simulink model "AC_base_1_VSM_2_22a"  (R2022a)
settings: Solver=ode3  StartTime=0.0  StopTime=8  FixedStep=HWSampleTime  RelTol=1e-3
undefined symbols (not defined in the file): ControlSampleTime, DiscIntNeverNeededParam, HWSampleTime, Ipwm_back, Ipwm_off, LCL, Manage, Oversample, Param, scaling_factor, SM, Ts, V_DC, VSMCTRL
libraries: fl_lib x100, nesl_utility x63, simulink x38, FriedrichLibrary x38, ee_lib x20, simulink_extras x14, TriphaseHardwaremodule x12, spsEdgeDetectorLib x2, StateMachines x2, slpidlib x2, spsPower3phInstantaneousLib x1
(part 5 of 7)

== system AC_base_1_VSM_2_22a/Variant Subsystem3/VSM/VSM1/VSM/CONTROL/VSMOC1 ==
  Manage : Inport
  Meas : Inport  Port=2
  u_inv_dq : Inport  Port=3
  Bus Selector1 : BusSelector  OutputSignals=enable_VSM.enable_ctrl,Param.VSM,enable_VSM.enable_inertia,sp_VSM
  Bus Selector11 : BusSelector  OutputSignals=phi
  Bus Selector2 : BusSelector  OutputSignals=PQ,PLL,u_cap.u_cap_dq0
  Selector : Selector  InputPortWidth=3  IndexOptions=Index vector (dialog)  Indices=[1 2]  OutputSizes=1
  Switch : Switch  Criteria=u2 ~= 0  SaturateOnIntegerOverflow=off  InputSameDT=off
  VSMOC : Subsystem
  phi_rad : Outport  VectorParamsAs1DForOutWhenUnconnected=off
  sp_u_inv_dq : Outport  Port=2  InitialOutput=[1 0]  VectorParamsAs1DForOutWhenUnconnected=off
  VSMdiag : Outport  Port=3  VectorParamsAs1DForOutWhenUnconnected=off
  wires:
  Bus Selector11/1 -> Switch/3  "<phi>"
  VSMOC/1(phi_rad) -> Switch/1
  VSMOC/3(VSMdiag) -> VSMdiag/1
  VSMOC/2(sp_u_inv_dq) -> sp_u_inv_dq/1
  Switch/1 -> phi_rad/1
  Manage/1 -> Bus Selector1/1
  Bus Selector1/1 -> VSMOC/Enable, Switch/2  "<enable_ctrl>"
  Meas/1 -> Bus Selector2/1
  Bus Selector2/2 -> VSMOC/5(PLL), Bus Selector11/1  "<PLL>"
  Bus Selector1/2 -> VSMOC/1(Param)  "<VSM>"
  Bus Selector1/3 -> VSMOC/2(enable_inertia)  "<enable_inertia>"
  Bus Selector1/4 -> VSMOC/3(sp_VSM)  "<sp_VSM>"
  u_inv_dq/1 -> VSMOC/6(u_inv_dq)
  Bus Selector2/3 -> Selector/1  "<u_cap_dq0>"
  Selector/1 -> VSMOC/7(u_cap_dq1)
  Bus Selector2/1 -> VSMOC/4(PQ_meas)  "<PQ>"

== system AC_base_1_VSM_2_22a/Variant Subsystem3/VSM/VSM1/VSM/CONTROL/Virtual Circuit mit R und L ==
  Param : Inport
  Reset : Inport  Port=2
  i_dq0 : Inport  Port=3
  Phi : Inport  Port=4
  Bus Selector : BusSelector  OutputSignals=R1,L1
  Bus Selector1 : BusSelector  OutputSignals=R1t,tauR,L1t,tauL
  Current Predictor : Subsystem  Commented=on
  L_Matrix : Gain  Gain=[0 -1 0;1 0 0; 0 0 0]
  L_Matrix1 : Gain  Gain=[0 -1 0;1 0 0; 0 0 0]
  PT1 : Subsystem  mask{K=1, Init=0, Ts=ControlSampleTime}
      mask prompts: K "Gain"; Init "Initial input"; Ts "Sample time"
      mask DialogControl DescGroupVar Prompt: PT1 discrete
      mask DialogControl DescTextVar Prompt: Simple discrete PT1
      mask Display:
      | text(0.5,0.5,get_param(gcb,'K'),'HorizontalAlignment','center','VerticalAlignment','Bottom')
      | text(0.5,0.5,'1 + s.tau','HorizontalAlignment','center','VerticalAlignment','Top')
      | plot([0.3 0.7],[0.5 0.5])
  PT2 : Subsystem  mask{K=1, Init=0, Ts=ControlSampleTime}
      mask prompts: K "Gain"; Init "Initial input"; Ts "Sample time"
      mask DialogControl DescGroupVar Prompt: PT1 discrete
      mask DialogControl DescTextVar Prompt: Simple discrete PT1
      mask Display:
      | text(0.5,0.5,get_param(gcb,'K'),'HorizontalAlignment','center','VerticalAlignment','Bottom')
      | text(0.5,0.5,'1 + s.tau','HorizontalAlignment','center','VerticalAlignment','Top')
      | plot([0.3 0.7],[0.5 0.5])
  "Param " : InportShadow
  Phi1 : InportShadow  Port=4
  Product : Product  Multiplication=Matrix(*)
  Product1 : Product  Multiplication=Matrix(*)
  Product2 : Product  Multiplication=Matrix(*)
  R_Matrix : Gain  Gain=[1 0 0;0 1 0; 0 0 0]
  R_Matrix1 : Gain  Gain=[1 0 0;0 1 0; 0 0 0]
  Reset1 : InportShadow  Port=2
  Sum : Sum  Inputs=++|
  Sum1 : Sum  Inputs=++|
  Sum2 : Sum  Inputs=|++
  " u_dq0" : Outport
  wires:
  Param/1 -> Bus Selector/1
  Bus Selector/1 -> R_Matrix/1  "<R1>"
  i_dq0/1 -> Product/2, PT2/1(U), PT1/1(U)
  Bus Selector/2 -> L_Matrix/1  "<L1>"
  L_Matrix/1 -> Sum/1
  R_Matrix/1 -> Sum/2
  Sum/1 -> Product/1
  "Param "/1 -> Bus Selector1/1
  R_Matrix1/1 -> Product1/1
  Product1/1 -> Sum1/1
  Bus Selector1/1 -> R_Matrix1/1  "<R1t>"
  Bus Selector1/4 -> PT2/2(tau)  "<tauL>"
  Bus Selector1/2 -> PT1/2(tau)  "<tauR>"
  Bus Selector1/3 -> L_Matrix1/1  "<L1t>"
  L_Matrix1/1 -> Product2/1
  Product2/1 -> Sum1/2
  Sum2/1 -> " u_dq0"/1
  PT1/1(Y) -> Product1/2
  Phi/1 -> PT1/4(Phi)
  Phi1/1 -> PT2/4(Phi)
  Reset/1 -> PT1/3(Reset)
  Reset1/1 -> PT2/3(Reset)
  PT2/1(Y) -> Product2/2
  Product/1 -> Sum2/1

== system AC_base_1_VSM_2_22a/Variant Subsystem3/VSM/VSM1/VSM/CONTROL/Virtual Circuit1 ==
  Param : Inport
  Reset : Inport  Port=2
  i_dq0 : Inport  Port=3
  Phi : Inport  Port=4
  Bus Selector : BusSelector  OutputSignals=R1,L1
  Bus Selector1 : BusSelector  OutputSignals=R1t,tauR,L1t,tauL
  Current Predictor : Subsystem  Commented=on
  L_Matrix : Gain  Gain=[0 -1 0;1 0 0; 0 0 0]
  L_Matrix1 : Gain  Gain=[0 -1 0;1 0 0; 0 0 0]
  PT1 : Subsystem  mask{K=1, Init=0, Ts=ControlSampleTime}
      mask prompts: K "Gain"; Init "Initial input"; Ts "Sample time"
      mask DialogControl DescGroupVar Prompt: PT1 discrete
      mask DialogControl DescTextVar Prompt: Simple discrete PT1
      mask Display:
      | text(0.5,0.5,get_param(gcb,'K'),'HorizontalAlignment','center','VerticalAlignment','Bottom')
      | text(0.5,0.5,'1 + s.tau','HorizontalAlignment','center','VerticalAlignment','Top')
      | plot([0.3 0.7],[0.5 0.5])
  PT2 : Subsystem  Commented=on  mask{K=1, Init=0, Ts=ControlSampleTime}
      mask prompts: K "Gain"; Init "Initial input"; Ts "Sample time"
      mask DialogControl DescGroupVar Prompt: PT1 discrete
      mask DialogControl DescTextVar Prompt: Simple discrete PT1
      mask Display:
      | text(0.5,0.5,get_param(gcb,'K'),'HorizontalAlignment','center','VerticalAlignment','Bottom')
      | text(0.5,0.5,'1 + s.tau','HorizontalAlignment','center','VerticalAlignment','Top')
      | plot([0.3 0.7],[0.5 0.5])
  "Param " : InportShadow
  Phi1 : InportShadow  Port=4
  Product : Product  Multiplication=Matrix(*)
  Product1 : Product  Multiplication=Matrix(*)
  Product2 : Product  Commented=on  Multiplication=Matrix(*)
  Product3 : Product  Multiplication=Matrix(*)
  R_Matrix : Gain  Gain=[1 0 0;0 1 0; 0 0 0]
  R_Matrix1 : Gain  Gain=[1 0 0;0 1 0; 0 0 0]
  Reset1 : InportShadow  Port=2
  Scope : Scope  NumInputPorts=2
  Scope1 : Scope
  Sum : Sum  Inputs=++|
  Sum1 : Sum  Inputs=++|
  Sum2 : Sum  Inputs=|++
  " u_dq0" : Outport
  wires:
  Param/1 -> Bus Selector/1
  Bus Selector/1 -> R_Matrix/1  "<R1>"
  i_dq0/1 -> PT2/1(U), PT1/1(U), Product3/2, Product/2
  Bus Selector/2 -> L_Matrix/1  "<L1>"
  L_Matrix/1 -> Sum/1
  R_Matrix/1 -> Product3/1, Sum/2
  Sum/1 -> Product/1
  "Param "/1 -> Bus Selector1/1
  Product/1 -> Sum2/1
  R_Matrix1/1 -> Product1/1
  Product1/1 -> Scope/2, Sum1/1
  Bus Selector1/1 -> R_Matrix1/1  "<R1t>"
  Bus Selector1/4 -> PT2/2(tau)  "<tauL>"
  Bus Selector1/2 -> PT1/2(tau)  "<tauR>"
  Bus Selector1/3 -> L_Matrix1/1  "<L1t>"
  L_Matrix1/1 -> Product2/1
  PT2/1(Y) -> Product2/2
  Product2/1 -> Scope1/1, Sum1/2
  Sum1/1 -> Sum2/2
  Sum2/1 -> " u_dq0"/1
  PT1/1(Y) -> Product1/2
  Phi1/1 -> PT2/4(Phi)
  Reset/1 -> PT1/3(Reset)
  Reset1/1 -> PT2/3(Reset)
  Product3/1 -> Scope/1

== system AC_base_1_VSM_2_22a/Variant Subsystem3/VSM/VSM1/VSM/CONTROL/active_damping ==
  enable_damp_dq : Inport
  Reset : Inport  Port=2
  u_dq0 : Inport  Port=3
  Phi : Inport  Port=4
  Bus Selector : BusSelector  OutputSignals=Damp_dq,Damp_dq,Damp_CM,OmLead,OmLag
  Integrator (inertia) : DiscreteIntegrator  gainval=1  ExternalReset=rising  InitialConditionSource=external  InitialCondition=1  SampleTime=ControlSampleTime  ICPrevOutput=DiscIntNeverNeededParam  ICPrevScaledInput=DiscIntNeverNeededParam
  Mux : Mux  Inputs=3
  Product{,1..3} (4 alike) : Product
  Sum : Sum  Inputs=|+-
  Sum2 : Sum  Inputs=++|
  Unit Delay2 : UnitDelay  InitialCondition=[0 0 0]  SampleTime=ControlSampleTime  HasFrameUpgradeWarning=on
  dq0->ab0 phi : FriedrichLibrary/Transformations/dq0->ab0 phi  SystemSampleTime=-1  VariantActivationTime=update diagram  Latency=0  AutoFrameSizeCalculation=off
  damp_dq0 : Outport  VectorParamsAs1DForOutWhenUnconnected=off
  wires:
  Product2/1 -> Sum/1
  Integrator (inertia)/1 -> Unit Delay2/1, Sum2/2
  Product3/1 -> Sum/2
  Sum2/1 -> Product3/1, Product1/2
  Sum/1 -> Integrator (inertia)/1
  enable_damp_dq/1 -> Bus Selector/1
  Bus Selector/1 -> Mux/1  "<Damp_dq>"
  Bus Selector/2 -> Mux/2  "<Damp_dq>"
  Bus Selector/3 -> Mux/3  "<Damp_CM>"
  u_dq0/1 -> Product/2
  Product/1 -> Sum2/1, Product2/2
  Mux/1 -> Product1/1, Product/1  "enable"
  Product1/1 -> damp_dq0/1
  Phi/1 -> dq0->ab0 phi/2
  Reset/1 -> Integrator (inertia)/2
  Unit Delay2/1 -> dq0->ab0 phi/1
  dq0->ab0 phi/1 -> Integrator (inertia)/3
  Bus Selector/4 -> Product2/1  "<OmLead>"
  Bus Selector/5 -> Product3/2  "<OmLag>"

== system AC_base_1_VSM_2_22a/Variant Subsystem3/VSM/VSM1/VSM/CONTROL/dq0 to duty ==
  phi_rad : Inport
  u_dq0 : Inport  Port=2
  u_dc : Inport  Port=3
  Bias : Bias  Bias=Ctrl.PWM.tauT*Ctrl.PU.omegab  SaturateOnIntegerOverflow=off
  Bus Creator3 : BusCreator  Inputs=2
  Divide : Product  Inputs=*/
  Gain : Gain  Gain=eye(NrChannels,3)  Multiplication=Matrix(K*u)
  Modulation : FriedrichLibrary/Transformations/Modulation  Method=Sine Modulation  Ts=ControlSampleTime
  SMA : FriedrichLibrary/Discrete Stuff/SMA  n_samples=1/ControlSampleTime/100  init_out=0
  Saturation : Saturate  UpperLimit=inf  LowerLimit=1
  Signal Specification1 : SignalSpecification
  dq0->ab0 phi : FriedrichLibrary/Transformations/dq0->ab0 phi  SystemSampleTime=-1  VariantActivationTime=update diagram  Latency=0  AutoFrameSizeCalculation=off
  d : Outport  VectorParamsAs1DForOutWhenUnconnected=off
  pwmDiag : Outport  Port=2  VectorParamsAs1DForOutWhenUnconnected=off
  wires:
  phi_rad/1 -> Bus Creator3/2, Bias/1  "phi"
  u_dq0/1 -> dq0->ab0 phi/1
  Divide/1 -> Modulation/1  "ab0 norm"
  dq0->ab0 phi/1 -> Divide/1
  Modulation/1 -> Gain/1
  Bias/1 -> dq0->ab0 phi/2
  u_dc/1 -> Saturation/1
  Bus Creator3/1 -> pwmDiag/1  "pwmDiag"
  Gain/1 -> Bus Creator3/1, Signal Specification1/1  "pwm"
  Signal Specification1/1 -> d/1
  Saturation/1 -> SMA/1
  SMA/1 -> Divide/2

== system AC_base_1_VSM_2_22a/Variant Subsystem3/VSM/VSM1/VSM/CONTROL/i_dq_ctrl ==
  note: Inrouting
  note: Outrouting
  note: PI Control
  Param : Inport
  enable_cc : Inport  Port=2
  sp_cc : Inport  Port=3
  ms_i_inv_dq : Inport  Port=4
  u_ff_dq : Inport  Port=5
  u_inv_dq : Inport  Port=6
  Enable : EnablePort  StatesWhenEnabling=reset
  Bus Creator2 : BusCreator  Inputs=4
  Bus Selector13 : BusSelector  OutputSignals=init_u_inv
  Constant : Constant
  Demux : Demux  Outputs=2
  From1 : From  Commented=on  GotoTag=initU
  Gain1 : Gain  Commented=on  Gain=Kff
  Gain2 : Gain  Gain=L_inv
  Gain4 : Gain  Gain=[0 -1;1 0]  Multiplication=Matrix(K*u)
  Gain5 : Gain  Commented=on  Gain=1-Kff
  Mux : Mux  Inputs=2
  PI : Subsystem
  Product : Product
  Product1 : Product
  Product2 : Product
  Scope : Scope  NumInputPorts=3
  Step : Step  Time=8  Before=1  After=0  SampleTime=0
  Sum1 : Sum  Inputs=+++
  Sum2 : Sum  Commented=on  Inputs=|+-
  Sum3 : Sum  Inputs=|+-
  Switch1 : Switch  Commented=on  Criteria=u2 > Threshold  SaturateOnIntegerOverflow=off  InputSameDT=off
  sp_u_inv_dq : Outport  VectorParamsAs1DForOutWhenUnconnected=off
  CCdiag : Outport  Port=2  VectorParamsAs1DForOutWhenUnconnected=off
  wires:
  Switch1/1 -> Sum2/1
  Gain4/1 -> Gain2/1
  Gain2/1 -> Sum2/2  "dq decouple"
  From1/1 -> Switch1/2
  Sum1/1 -> Scope/1, Product/2
  u_inv_dq/1 -> Switch1/1
  [Enable] -> PI/Enable
  Sum3/1 -> Demux/1
  sp_cc/1 -> [sp_i_dq], Sum3/1
  Param/1 -> Bus Selector13/1
  Bus Selector13/1 -> [initU]  "<init_u_inv>"
  [Enable] -> Product/1
  [sp_u_dq] -> Bus Creator2/3  "sp_u_dq"
  enable_cc/1 -> [Enable]  "enable_cc"
  [Enable] -> Bus Creator2/4  "enable_cc"
  Bus Creator2/1 -> CCdiag/1
  [sp_i_dq] -> Bus Creator2/1  "sp_i_dq"
  [i_dq] -> Bus Creator2/2  "i_dq"
  u_ff_dq/1 -> Scope/2, PI/2(u0), Gain1/1, Gain5/1
  Gain5/1 -> Switch1/3
  Product/1 -> sp_u_inv_dq/1, [sp_u_dq]
  ms_i_inv_dq/1 -> [i_dq], Sum3/2, Gain4/1
  Mux/1 -> PI/1(di)
  Demux/2 -> Product1/1
  Product1/1 -> Mux/2
  Product2/1 -> Mux/1
  Demux/1 -> Product2/1
  Constant/1 -> Product2/2, Product1/2
  PI/1(u) -> Sum1/1  "pi"

== system AC_base_1_VSM_2_22a/Variant Subsystem3/VSM/VSM1/VSM/MANAGEMENT/Subsystem1 ==
  i_inv_ab : Inport
  <i_inv_dq0> : Inport  Port=2
  <u_cap_ab0> : Inport  Port=3
  <PQ_out> : Inport  Port=4
  enable : Inport  Port=5
  i_out_ab : Inport  Port=6
  "AL brechen AL nicht mit FCN lösbar " : Memory
  Compare To Constant : simulink/Logic and Bit Operations/Compare To Constant  relop===  const=0  OutDataTypeStr=boolean
  Complex to Magnitude-Angle : ComplexToMagnitudeAngle
  Demux : Demux  Outputs=2
  Divide : Product  Inputs=*/
  Enabled Subsystem : Subsystem  TreatAsAtomicUnit=on
  Math Function1 : Math  Operator=square  SignedPower=on
  Math Function2 : Math  Operator=square  SignedPower=on
  Math Function3 : Math  Operator=square  SignedPower=on
  Max : MinMax  Function=max  Inputs=2
  Real-Imag to Complex : RealImagToComplex
  Scope : Scope  NumInputPorts=2
  Selector2 : Selector  InputPortWidth=3  IndexOptions=Index vector (dialog)  Indices=[1 2]  OutputSizes=1
  Sqrt1 : Sqrt
  Sqrt2 : Sqrt
  Sqrt3 : Sqrt
  Subsystem : Subsystem
  Sum of Elements1 : Sum  Inputs=+
  Sum of Elements2 : Sum  Inputs=+
  Sum of Elements3 : Sum  Inputs=+
  Transport Delay : TransportDelay  DelayTime=0.1
  Transport Delay1 : TransportDelay  DelayTime=0.1
  Unit Delay : UnitDelay  SampleTime=ControlSampleTime  HasFrameUpgradeWarning=on
  Unit Delay1 : UnitDelay  SampleTime=ControlSampleTime  HasFrameUpgradeWarning=on
  CC : Outport
  sp_CC : Outport  Port=2
  wires:
  Sum of Elements1/1 -> Sqrt2/1
  Selector2/1 -> Math Function2/1
  Math Function1/1 -> Sum of Elements1/1
  Sum of Elements2/1 -> Sqrt1/1
  "AL brechen AL nicht mit FCN lösbar "/1 -> Subsystem/1(i_inv)
  Sqrt1/1 -> Subsystem/4(U_cap), Divide/2
  Math Function2/1 -> Sum of Elements2/1
  <u_cap_ab0>/1 -> Selector2/1
  <i_inv_dq0>/1 -> "AL brechen AL nicht mit FCN lösbar "/1
  Subsystem/1(i_sp) -> sp_CC/1  "sp_CC"
  i_inv_ab/1 -> Math Function1/1
  Subsystem/2(CC) -> CC/1
  <PQ_out>/1 -> Divide/1, Subsystem/2(PQ_out)
  enable/1 -> Subsystem/Enable
  Compare To Constant/1 -> Enabled Subsystem/Enable
  Enabled Subsystem/1(i abs_pre) -> Scope/1, Unit Delay/1
  Subsystem/3(set) -> Compare To Constant/1
  Transport Delay/1 -> Enabled Subsystem/1(i_abs)
  Unit Delay/1 -> Subsystem/6(i abs_pre)
  Enabled Subsystem/2(i_pq_pre) -> Unit Delay1/1, Scope/2
  Unit Delay1/1 -> Subsystem/5(PQ_pre)
  Transport Delay1/1 -> Enabled Subsystem/2(i_pq)
  Math Function3/1 -> Sum of Elements3/1
  Sum of Elements3/1 -> Sqrt3/1
  i_out_ab/1 -> Math Function3/1
  Sqrt3/1 -> Max/1
  Sqrt2/1 -> Max/2, Transport Delay/1
  Max/1 -> Subsystem/3(iabs)
  Demux/1 -> Real-Imag to Complex/1
  Demux/2 -> Real-Imag to Complex/2
  Divide/1 -> Demux/1, Transport Delay1/1
  Real-Imag to Complex/1 -> Complex to Magnitude-Angle/1
  Complex to Magnitude-Angle/2 -> Subsystem/7(angle_i)

== system AC_base_1_VSM_2_22a/Variant Subsystem3/VSM/VSM1/VSM/MANAGEMENT/current_watchdog ==
  |i| set : Inport
  |i| reset : Inport  Port=2
  i_ab : Inport  Port=3
  sp_gain : Inport  Port=4
  PQ : Inport  Port=5
  i_inv : Inport  Port=6
  active_current_watchdog : EnablePort  StatesWhenEnabling=reset
  Divide : Product  Inputs=/**
  MATLAB Function : MATLAB Function  Commented=on  TreatAsAtomicUnit=on
  Math Function1 : Math  Operator=square  SignedPower=on
  Math Function2 : Math  Operator=square  SignedPower=on
  Math Function3 : Math  Operator=square  SignedPower=on
  Relational Operator : RelationalOperator  Operator=<=  OutDataTypeStr=boolean  InputSameDT=off
  Relational Operator1 : RelationalOperator  Operator=<=  OutDataTypeStr=boolean  InputSameDT=off
  S-R Flip-Flop1 : simulink_extras/Flip Flops/S-R Flip-Flop  initial_condition=0
  Scope : Scope  NumInputPorts=3
  Scope1 : Scope
  Sum of Elements1 : Sum  Inputs=+
  Terminator1 : Terminator
  enable_cc : Outport  VectorParamsAs1DForOutWhenUnconnected=off
  sp_gain_wd : Outport  Port=2  VectorParamsAs1DForOutWhenUnconnected=off
  wires:
  Math Function2/1 -> Relational Operator/1, MATLAB Function/2(set)
  i_ab/1 -> Math Function1/1
  Sum of Elements1/1 -> Relational Operator1/1, MATLAB Function/1(abs), Relational Operator/2
  Math Function1/1 -> Sum of Elements1/1
  Relational Operator1/1 -> S-R Flip-Flop1/2
  S-R Flip-Flop1/2 -> Terminator1/1
  Math Function3/1 -> Relational Operator1/2
  |i| reset/1 -> Divide/2, Math Function3/1
  |i| set/1 -> Divide/1, Math Function2/1
  sp_gain/1 -> Divide/3
  MATLAB Function/1(CC) -> enable_cc/1, Scope/1
  MATLAB Function/2(i) -> sp_gain_wd/1
  PQ/1 -> Scope1/1, MATLAB Function/3(p)
  i_inv/1 -> MATLAB Function/4(i_inv)

== system AC_base_1_VSM_2_22a/Variant Subsystem3/VSM/VSM1/VSM/MANAGEMENT/sp_VSM ==
  EnableRateLimit : Inport
  CMD : Inport  Port=2
  MEAS : Inport  Port=3
  Bus Creator : BusCreator  Inputs=3
  Bus Selector1 : BusSelector  OutputSignals=u_out.u_out_ab0
  Bus Selector6 : BusSelector  OutputSignals=Param.VSM.sp_f,Param.VSM.sp_E,Param.VSM.sp_PQ,Param.VSM.sp_PQ_limit
  "CMD " : InportShadow  Port=2
  E(PQ) : Subsystem
  PQ(U) Limit : Subsystem
  RateLimit : Subsystem
  Saturation : Saturate  UpperLimit=1  LowerLimit=-1
  sp_VSM : Outport  VectorParamsAs1DForOutWhenUnconnected=off
  wires:
  E(PQ)/1(sp_E) -> Bus Creator/2  "sp_E"
  Bus Selector6/2 -> E(PQ)/1(E)  "<sp_E>"
  Bus Selector6/3 -> Saturation/1  "<sp_PQ>"
  EnableRateLimit/1 -> RateLimit/Enable  "ENABLED"
  RateLimit/1(PQslow) -> E(PQ)/3(sp_PQ), PQ(U) Limit/1(sp_PQ)
  Bus Selector1/1 -> PQ(U) Limit/3(u_out)  "<u_out_ab0>"
  Bus Selector6/4 -> PQ(U) Limit/2(enable)  "<sp_PQ_limit>"
  PQ(U) Limit/1(sp_PQ_limit) -> Bus Creator/3  "sp_PQ"
  CMD/1 -> Bus Selector6/1
  MEAS/1 -> Bus Selector1/1
  Bus Selector6/1 -> Bus Creator/1  "<sp_f>"
  Bus Creator/1 -> sp_VSM/1
  "CMD "/1 -> E(PQ)/2(cmd)
  Saturation/1 -> RateLimit/1(PQ)

== system AC_base_1_VSM_2_22a/Variant Subsystem3/VSM/VSM1/VSM/Meas/SI -> pu ==
  MeasIn : Inport
  Bus Creator1 : BusCreator  Inputs=5
  Bus Selector : BusSelector  OutputSignals=meas_u_out,meas_i_out,meas_i_inverter,meas_u_dc,meas_u_cap
  Normalize : Gain  Gain=1/PU.Ub  OutDataTypeStr=double  RndMeth=Round
  Normalize1 : Gain  Gain=1/PU.Ib  OutDataTypeStr=double  RndMeth=Round
  Normalize2 : Gain  Gain=1/PU.Ib  OutDataTypeStr=double  RndMeth=Round
  Normalize3 : Gain  Gain=1/PU.Ub  OutDataTypeStr=double  RndMeth=Round
  Normalize4 : Gain  Gain=1/PU.Ub/2  OutDataTypeStr=double  RndMeth=Round
  MeasOut : Outport  VectorParamsAs1DForOutWhenUnconnected=off
  wires:
  Normalize3/1 -> Bus Creator1/5  "meas_u_cap"
  Bus Selector/5 -> Normalize3/1  "<meas_u_cap>"
  Bus Selector/4 -> Normalize4/1  "<meas_u_dc>"
  Bus Selector/3 -> Normalize1/1  "<meas_i_inverter>"
  Bus Selector/2 -> Normalize2/1  "<meas_i_out>"
  Bus Selector/1 -> Normalize/1  "<meas_u_out>"
  Bus Creator1/1 -> MeasOut/1
  Normalize4/1 -> Bus Creator1/4  "meas_vol_dc"
  Normalize2/1 -> Bus Creator1/2  "meas_i_out"
  Normalize1/1 -> Bus Creator1/3  "meas_i_inverter"
  Normalize/1 -> Bus Creator1/1  "meas_u_out"
  MeasIn/1 -> Bus Selector/1

== system AC_base_1_VSM_2_22a/Variant Subsystem3/VSM/VSM1/VSM/Meas/meas_i_inv ==
  abc : Inport
  phi : Inport  Port=2
  Bus Creator1 : BusCreator  Inputs=3
  PhN->ab2 : FriedrichLibrary/Transformations/PhN->ab0  SystemSampleTime=-1  VariantActivationTime=update diagram  Latency=0  AutoFrameSizeCalculation=off
  ab0->dq0-faster : FriedrichLibrary/Transformations/ab0->dq0-faster  SystemSampleTime=-1  VariantActivationTime=update diagram  Latency=0  AutoFrameSizeCalculation=off
  i_inv_x : Outport  VectorParamsAs1DForOutWhenUnconnected=off
  wires:
  ab0->dq0-faster/1 -> Bus Creator1/3  "i_inv_dq0"
  PhN->ab2/1 -> Bus Creator1/2, ab0->dq0-faster/1  "i_inv_ab0"
  abc/1 -> Bus Creator1/1, PhN->ab2/1  "i_inv_abc"
  phi/1 -> ab0->dq0-faster/2
  Bus Creator1/1 -> i_inv_x/1

== system AC_base_1_VSM_2_22a/Variant Subsystem3/VSM/VSM1/VSM/Meas/meas_i_out ==
  abc : Inport
  phi : Inport  Port=2
  Bus Creator1 : BusCreator  Inputs=3
  PhN->ab2 : FriedrichLibrary/Transformations/PhN->ab0  SystemSampleTime=-1  VariantActivationTime=update diagram  Latency=0  AutoFrameSizeCalculation=off
  ab0->dq0-faster : FriedrichLibrary/Transformations/ab0->dq0-faster  SystemSampleTime=-1  VariantActivationTime=update diagram  Latency=0  AutoFrameSizeCalculation=off
  i_out_x : Outport  VectorParamsAs1DForOutWhenUnconnected=off
  wires:
  ab0->dq0-faster/1 -> Bus Creator1/3  "i_out_dq0"
  PhN->ab2/1 -> Bus Creator1/2, ab0->dq0-faster/1  "i_out_ab0"
  abc/1 -> Bus Creator1/1, PhN->ab2/1  "i_out_abc"
  phi/1 -> ab0->dq0-faster/2
  Bus Creator1/1 -> i_out_x/1

== system AC_base_1_VSM_2_22a/Variant Subsystem3/VSM/VSM1/VSM/Meas/meas_u_cap ==
  abc : Inport
  phi : Inport  Port=2
  Bus Creator1 : BusCreator  Inputs=3
  PhN->ab2 : FriedrichLibrary/Transformations/PhN->ab0  SystemSampleTime=-1  VariantActivationTime=update diagram  Latency=0  AutoFrameSizeCalculation=off
  ab0->dq0-faster : FriedrichLibrary/Transformations/ab0->dq0-faster  SystemSampleTime=-1  VariantActivationTime=update diagram  Latency=0  AutoFrameSizeCalculation=off
  u_cap_x : Outport  VectorParamsAs1DForOutWhenUnconnected=off
  wires:
  Bus Creator1/1 -> u_cap_x/1
  phi/1 -> ab0->dq0-faster/2
  abc/1 -> PhN->ab2/1, Bus Creator1/1  "u_cap_abc"
  PhN->ab2/1 -> ab0->dq0-faster/1, Bus Creator1/2  "u_cap_ab0"
  ab0->dq0-faster/1 -> Bus Creator1/3  "u_cap_dq0"

== system AC_base_1_VSM_2_22a/Variant Subsystem3/VSM/VSM1/VSM/Meas/meas_u_out ==
  abc : Inport
  phi : Inport  Port=2
  Bus Creator1 : BusCreator  Inputs=3
  PhN->ab2 : FriedrichLibrary/Transformations/PhN->ab0  SystemSampleTime=-1  VariantActivationTime=update diagram  Latency=0  AutoFrameSizeCalculation=off
  ab0->dq0-faster : FriedrichLibrary/Transformations/ab0->dq0-faster  SystemSampleTime=-1  VariantActivationTime=update diagram  Latency=0  AutoFrameSizeCalculation=off
  u_out_x : Outport  VectorParamsAs1DForOutWhenUnconnected=off
  wires:
  Bus Creator1/1 -> u_out_x/1
  phi/1 -> ab0->dq0-faster/2
  abc/1 -> PhN->ab2/1, Bus Creator1/1  "u_out_abc"
  PhN->ab2/1 -> ab0->dq0-faster/1, Bus Creator1/2  "u_out_ab0"
  ab0->dq0-faster/1 -> Bus Creator1/3  "u_out_dq0"

== system AC_base_1_VSM_2_22a/Variant Subsystem3/VSM/VSM1/command_center/cmd_VSM/Current Control ==
  note: else: init with u cap
  Bus Creator6 : BusCreator  Inputs=5
  Bus Creator7 : BusCreator  Inputs=3
  Init with u_inv [0/1] : Constant  Value=VSMCTRL.CC.init_uinv
  activate : Constant  Value=VSMCTRL.CC.activate
  external_stop_cc1 : Constant  Value=0
  external_stop_cc4 : Constant  Value=0
  i_reset_abs : Constant  Value=VSMCTRL.CC.i_reset
  i_set_abs : Constant  Value=VSMCTRL.CC.i_set
  i_sp_gain : Constant  Value=VSMCTRL.CC.i_sp_gain
  Current Control : Outport  VectorParamsAs1DForOutWhenUnconnected=off
  wires:
  activate/1 -> Bus Creator7/1  "activate"
  i_reset_abs/1 -> Bus Creator7/3  "abs_i_reset"
  Bus Creator7/1 -> Bus Creator6/5  "watchdog"
  external_stop_cc4/1 -> Bus Creator6/2  "ex_start_cc"
  i_set_abs/1 -> Bus Creator7/2  "abs_i_set"
  i_sp_gain/1 -> Bus Creator6/4  "i_sp_gain"
  external_stop_cc1/1 -> Bus Creator6/3  "ex_stop_cc"
  Init with u_inv [0/1]/1 -> Bus Creator6/1  "init_u_inv"
  Bus Creator6/1 -> Current Control/1  "CC"

== system AC_base_1_VSM_2_22a/Variant Subsystem3/VSM/VSM1/command_center/cmd_VSM/Damping ==
  Bus Creator5 : BusCreator  Inputs=4
  EnableDamp_CM [0/1] : Constant  Value=VSMCTRL.VTFF.EnableCM
  EnableDamp_dq [0/1] : Constant  Value=VSMCTRL.VTFF.EnableDQ
  Omega Lag : Constant  Value=VSMCTRL.VTFF.OmLag
  Omega Lead : Constant  Value=VSMCTRL.VTFF.OmLead
  Damping : Outport  VectorParamsAs1DForOutWhenUnconnected=off
  wires:
  EnableDamp_CM [0/1]/1 -> Bus Creator5/2  "Damp_CM"
  EnableDamp_dq [0/1]/1 -> Bus Creator5/1  "Damp_dq"
  Bus Creator5/1 -> Damping/1
  Omega Lead/1 -> Bus Creator5/3  "OmLead"
  Omega Lag/1 -> Bus Creator5/4  "OmLag"

== system AC_base_1_VSM_2_22a/Variant Subsystem3/VSM/VSM1/command_center/cmd_VSM/Manage ==
  Bus Creator : BusCreator  Inputs=2
  connect : Constant
  enable : Constant
  Manage : Outport  VectorParamsAs1DForOutWhenUnconnected=off
  wires:
  Bus Creator/1 -> Manage/1
  connect/1 -> Bus Creator/1  "connect"
  enable/1 -> Bus Creator/2  "enable"

== system AC_base_1_VSM_2_22a/Variant Subsystem3/VSM/VSM1/command_center/cmd_VSM/Virtual Circuit ==
  Bus Creator9 : BusCreator  Inputs=7
  Virtual L1 : Constant  Value=VSMCTRL.VC.L1
  Virtual L1t : Constant  Value=VSMCTRL.VC.L1t
  Virtual R1 : Constant  Value=VSMCTRL.VC.R1
  Virtual R1t : Constant  Value=VSMCTRL.VC.R1t
  tau HP Slow : Constant  Value=VSMCTRL.VC.tauSlow
  tau Virtual L1 : Constant  Value=VSMCTRL.VC.tauL
  tau Virtual R1 : Constant  Value=VSMCTRL.VC.tauR
  Virtual Circuit : Outport  VectorParamsAs1DForOutWhenUnconnected=off
  wires:
  Virtual R1/1 -> Bus Creator9/1  "R1"
  Virtual R1t/1 -> Bus Creator9/2  "R1t"
  Virtual L1t/1 -> Bus Creator9/4  "L1t"
  Bus Creator9/1 -> Virtual Circuit/1
  Virtual L1/1 -> Bus Creator9/3  "L1"
  tau Virtual R1/1 -> Bus Creator9/5  "tauR"
  tau Virtual L1/1 -> Bus Creator9/6  "tauL"
  tau HP Slow/1 -> Bus Creator9/7  "tauS"

== system AC_base_1_VSM_2_22a/Variant Subsystem3/VSM/VSM1/command_center/cmd_VSM/Virtual Synchronous Machine ==
  note: 0 Dekaktiviert Init Tiefpass
  note: 0 Dekaktiviert Init Tiefpass
  Bus Creator3 : BusCreator  Inputs=12
  E(sp_PQ) : Constant  Value=VSMCTRL.SP.E_comp
  Ta : Constant  Value=VSMCTRL.VSM.Ta
  Ta1 : Constant  Value=VSMCTRL.VSM.kpf
  Ta2 : Constant  Value=VSMCTRL.VSM.kdf
  Ta3 : Constant  Value=VSMCTRL.VSM.ku
  Ta4 : Constant  Value=VSMCTRL.VSM.Tu
  Ta5 : Constant  Value=0
  Ta6 : Constant  Value=0
  sp_E [pu] : Constant  Value=VSMCTRL.SP.E
  sp_PQ [pu] : Constant  Value=VSMCTRL.SP.PQ
  sp_PQ(U) limit : Constant  Value=VSMCTRL.SP.PQU_lim
  sp_f [Hz] : Constant  Value=VSMCTRL.SP.f
  Virtual Synchronous Machine : Outport  VectorParamsAs1DForOutWhenUnconnected=off
  wires:
  sp_E [pu]/1 -> Bus Creator3/10  "sp_E"
  sp_PQ [pu]/1 -> Bus Creator3/9  "sp_PQ"
  sp_f [Hz]/1 -> Bus Creator3/8  "sp_f"
  sp_PQ(U) limit/1 -> Bus Creator3/11  "sp_PQ_limit"
  Ta/1 -> Bus Creator3/1  "Ta"
  Bus Creator3/1 -> Virtual Synchronous Machine/1
  Ta4/1 -> Bus Creator3/5  "Tu"
  Ta3/1 -> Bus Creator3/4  "ku"
  Ta2/1 -> Bus Creator3/3  "kdf"
  Ta1/1 -> Bus Creator3/2  "kpf"
  Ta6/1 -> Bus Creator3/7  "TPinit"
  Ta5/1 -> Bus Creator3/6  "Tuinit"
  E(sp_PQ)/1 -> Bus Creator3/12  "sp_E_comp"

== system AC_base_1_VSM_2_22a/Variant Subsystem1/VSM/Inverter AverageMdl LC SimScape2/Modul F30 fixed DC voltage Average SimScape/simscape_bridgefilter_aca/PWM Blocking1/Trigger Spike at new Control Sample ==
  Add : Sum  Inputs=+-
  Compare To Constant : simulink/Logic and Bit Operations/Compare To Constant  relop=~=  const=0  OutDataTypeStr=boolean
  Rate Transition : RateTransition  OutPortSampleTime=ControlSampleTime
  Rate Transition1 : RateTransition  OutPortSampleTime=ControlSampleTime
  Rate Transition2 : RateTransition  OutPortSampleTime=ControlSampleTime/Oversample
  S-R Flip-Flop1 : simulink_extras/Flip Flops/S-R Flip-Flop  initial_condition=1
  Unit Delay : UnitDelay  SampleTime=-1  HasFrameUpgradeWarning=on
  Unit Delay2 : UnitDelay  SampleTime=-1  HasFrameUpgradeWarning=on
  Unit Delay3 : UnitDelay  SampleTime=-1  HasFrameUpgradeWarning=on
  y : Outport
  wires:
  Rate Transition1/1 -> Unit Delay2/1
  Rate Transition/1 -> Unit Delay/1
  Unit Delay/1 -> S-R Flip-Flop1/2
  Add/1 -> Compare To Constant/1
  Compare To Constant/1 -> y/1
  Unit Delay3/1 -> Add/1
  Unit Delay2/1 -> S-R Flip-Flop1/1
  S-R Flip-Flop1/2 -> Rate Transition1/1
  Rate Transition2/1 -> Unit Delay3/1, Add/2
  S-R Flip-Flop1/1 -> Rate Transition/1, Rate Transition2/1

== system AC_base_1_VSM_2_22a/Variant Subsystem1/VSM/Inverter AverageMdl LC SimScape2/Modul F30 fixed DC voltage Average SimScape/simscape_bridgefilter_aca1/PWM Blocking1/Trigger Spike at new Control Sample ==
  Add : Sum  Inputs=+-
  Compare To Constant : simulink/Logic and Bit Operations/Compare To Constant  relop=~=  const=0  OutDataTypeStr=boolean
  Rate Transition : RateTransition  OutPortSampleTime=ControlSampleTime
  Rate Transition1 : RateTransition  OutPortSampleTime=ControlSampleTime
  Rate Transition2 : RateTransition  OutPortSampleTime=ControlSampleTime/Oversample
  S-R Flip-Flop1 : simulink_extras/Flip Flops/S-R Flip-Flop  initial_condition=1
  Unit Delay : UnitDelay  SampleTime=-1  HasFrameUpgradeWarning=on
  Unit Delay2 : UnitDelay  SampleTime=-1  HasFrameUpgradeWarning=on
  Unit Delay3 : UnitDelay  SampleTime=-1  HasFrameUpgradeWarning=on
  y : Outport
  wires:
  S-R Flip-Flop1/1 -> Rate Transition2/1, Rate Transition/1
  Rate Transition2/1 -> Add/2, Unit Delay3/1
  S-R Flip-Flop1/2 -> Rate Transition1/1
  Unit Delay2/1 -> S-R Flip-Flop1/1
  Unit Delay3/1 -> Add/1
  Compare To Constant/1 -> y/1
  Add/1 -> Compare To Constant/1
  Unit Delay/1 -> S-R Flip-Flop1/2
  Rate Transition/1 -> Unit Delay/1
  Rate Transition1/1 -> Unit Delay2/1

== system AC_base_1_VSM_2_22a/Variant Subsystem1/VSM/Inverter AverageMdl LC SimScape2/Modul F30 fixed DC voltage Average SimScape/simscape_bridgefilter_aca2/PWM Blocking1/Trigger Spike at new Control Sample ==
  Add : Sum  Inputs=+-
  Compare To Constant : simulink/Logic and Bit Operations/Compare To Constant  relop=~=  const=0  OutDataTypeStr=boolean
  Rate Transition : RateTransition  OutPortSampleTime=ControlSampleTime
  Rate Transition1 : RateTransition  OutPortSampleTime=ControlSampleTime
  Rate Transition2 : RateTransition  OutPortSampleTime=ControlSampleTime/Oversample
  S-R Flip-Flop1 : simulink_extras/Flip Flops/S-R Flip-Flop  initial_condition=1
  Unit Delay : UnitDelay  SampleTime=-1  HasFrameUpgradeWarning=on
  Unit Delay2 : UnitDelay  SampleTime=-1  HasFrameUpgradeWarning=on
  Unit Delay3 : UnitDelay  SampleTime=-1  HasFrameUpgradeWarning=on
  y : Outport
  wires:
  Rate Transition1/1 -> Unit Delay2/1
  Rate Transition/1 -> Unit Delay/1
  Unit Delay/1 -> S-R Flip-Flop1/2
  Add/1 -> Compare To Constant/1
  Compare To Constant/1 -> y/1
  Unit Delay3/1 -> Add/1
  Unit Delay2/1 -> S-R Flip-Flop1/1
  S-R Flip-Flop1/2 -> Rate Transition1/1
  Rate Transition2/1 -> Unit Delay3/1, Add/2
  S-R Flip-Flop1/1 -> Rate Transition/1, Rate Transition2/1

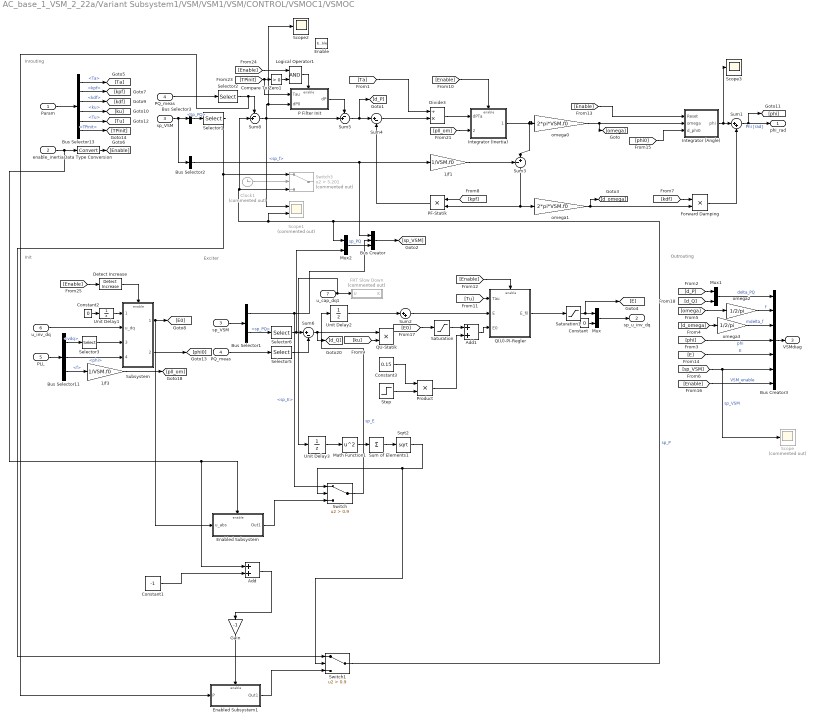
== system AC_base_1_VSM_2_22a/Variant Subsystem1/VSM/VSM1/VSM/CONTROL/VSMOC1/VSMOC ==
  note: Outrouting
  note: Init
  note: Exciter
  note: Inrouting
  Param : Inport
  enable_inertia : Inport  Port=2
  sp_VSM : Inport  Port=3
  PQ_meas : Inport  Port=4
  PLL : Inport  Port=5
  u_inv_dq : Inport  Port=6
  u_cap_dq1 : Inport  Port=7
  Enable : EnablePort  StatesWhenEnabling=reset
  1/f1 : Gain  Gain=1/VSM.f0
  1/f3 : Gain  Gain=1/VSM.f0
  Add : Sum
  Add1 : Sum
  Bus Creator : BusCreator  Inputs=3
  Bus Creator3 : BusCreator  Inputs=7
  Bus Selector1 : BusSelector  OutputSignals=sp_E,sp_PQ
  Bus Selector11 : BusSelector  OutputSignals=vdq,phi,f
  Bus Selector13 : BusSelector  OutputSignals=Ta,kpf,kdf,ku,Tu,TPinit
  Bus Selector2 : BusSelector  OutputSignals=sp_f
  Bus Selector3 : BusSelector  OutputSignals=sp_PQ
  Clock1 : Clock  Commented=on
  Compare To Zero1 : simulink/Logic and Bit Operations/Compare To Zero  relop=>  OutDataTypeStr=boolean
  Constant : Constant  Value=0
  Constant1 : Constant  Value=-1
  Constant2 : Constant  Value=0  SampleTime=ControlSampleTime
  Constant3 : Constant  Value=0.15
  Data Type Conversion : DataTypeConversion  SaturateOnIntegerOverflow=off  RndMeth=Floor
  Detect Increase : simulink/Logic and Bit Operations/Detect Increase  vinit=0.0  OutDataTypeStr=boolean
  Divide3 : Product  Inputs=/*
  Enabled Subsystem : Subsystem  TreatAsAtomicUnit=on
  Enabled Subsystem1 : Subsystem  TreatAsAtomicUnit=on
  FRT Slow Down : Subsystem  Commented=on
  Forward Damping : Product  Inputs=**
  Gain : Gain  Gain=-1
  Integrator (Angle) : Subsystem
  Integrator (Inertia) : Subsystem
  Logical Operator1 : Logic  AllPortsSameDT=off  OutDataTypeStr=boolean
  Math Function1 : Math  Operator=square  SignedPower=on
  Mux : Mux  Inputs=2
  Mux1 : Mux  Inputs=2
  Mux2 : Mux  Inputs=2
  P Filter Init : Subsystem
  PF-Statik : Product  Inputs=**
  "PQ_meas " : InportShadow  Port=4
  Product : Product
  Q(U)-PI-Regler : Subsystem
  QU-Statik : Product  Inputs=**
  Saturation : Saturate  UpperLimit=1.8  LowerLimit=0.8*0
  Saturation1 : Saturate  UpperLimit=2
  Scope : Scope  Commented=on
  Scope1 : Scope  Commented=on  NumInputPorts=2
  Scope2 : Scope
  Scope3 : Scope
  Selector1 : Selector  InputPortWidth=2  IndexOptions=Index vector (dialog)  Indices=1  OutputSizes=1
  Selector2 : Selector  InputPortWidth=2  IndexOptions=Index vector (dialog)  Indices=1  OutputSizes=1
  Selector3 : Selector  InputPortWidth=3  IndexOptions=Index vector (dialog)  Indices=[1 2]  OutputSizes=1
  Selector5 : Selector  InputPortWidth=2  IndexOptions=Index vector (dialog)  Indices=2  OutputSizes=1
  Selector6 : Selector  InputPortWidth=2  IndexOptions=Index vector (dialog)  Indices=2  OutputSizes=1
  Sqrt2 : Sqrt
  Step : Step  Time=2  After=0  SampleTime=0
  Subsystem : Subsystem
  Sum of Elements1 : Sum  Inputs=+
  Sum1 : Sum  Inputs=|++
  Sum2 : Sum  Inputs=|++
  Sum3 : Sum  Inputs=-+|
  Sum4 : Sum  Inputs=|+-
  Sum5 : Sum  Inputs=-+|
  Sum6 : Sum  Inputs=|+-
  Sum8 : Sum  Inputs=-+|
  Switch : Switch  Criteria=u2 > Threshold  Threshold=0.9  SaturateOnIntegerOverflow=off  InputSameDT=off
  Switch1 : Switch  Criteria=u2 > Threshold  Threshold=0.9  SaturateOnIntegerOverflow=off  InputSameDT=off
  Switch3 : Switch  Commented=on  Criteria=u2 > Threshold  Threshold=5.201  SaturateOnIntegerOverflow=off  InputSameDT=off
  Unit Delay1 : UnitDelay  InitialCondition=1  SampleTime=ControlSampleTime  HasFrameUpgradeWarning=on
  Unit Delay2 : UnitDelay  SampleTime=-1  HasFrameUpgradeWarning=on
  Unit Delay3 : UnitDelay  SampleTime=-1  HasFrameUpgradeWarning=on
  omega0 : Gain  Gain=2*pi*VSM.f0
  omega1 : Gain  Gain=2*pi*VSM.f0
  omega2 : Gain  Gain=1/2/pi
  omega3 : Gain  Gain=1/2/pi
  "sp_VSM " : InportShadow  Port=3
  phi_rad : Outport  VectorParamsAs1DForOutWhenUnconnected=off
  sp_u_inv_dq : Outport  Port=2  InitialOutput=[1 0]  VectorParamsAs1DForOutWhenUnconnected=off
  VSMdiag : Outport  Port=3  VectorParamsAs1DForOutWhenUnconnected=off
  wires:
  Bus Creator/1 -> [sp_VSM]
  Mux2/1 -> Bus Creator/3  "sp_PQ"
  Product/1 -> Add1/2
  Constant3/1 -> Product/1
  Step/1 -> Product/2
  Add1/1 -> Q(U)-PI-Regler/3(E0)
  Saturation/1 -> Add1/1
  Add/1 -> Gain/1
  Gain/1 -> Enabled Subsystem1/Enable
  Constant1/1 -> Add/2
  Selector1/1 -> Switch1/1, Switch3/1
  Q(U)-PI-Regler/1(E_fil) -> Saturation1/1
  Clock1/1 -> Switch3/2
  Switch1/1 -> Mux2/1, Switch3/3, Sum8/2, Scope1/2  "sp_P"
  Switch/1 -> Unit Delay2/1  "sp_E"
  Enabled Subsystem1/1(Out1) -> Switch1/3
  Subsystem/1(u_abs) -> [E0], Enabled Subsystem/1(u_abs)
  Enabled Subsystem/1(Out1) -> Switch/3
  enable_inertia/1 -> Data Type Conversion/1, Enabled Subsystem/Enable, Add/1
  Bus Selector1/1 -> Switch/1, Bus Creator/2  "<sp_E>"
  Math Function1/1 -> Sum of Elements1/1
  Unit Delay3/1 -> Math Function1/1
  Sum of Elements1/1 -> Sqrt2/1
  u_cap_dq1/1 -> FRT Slow Down/1(U), Unit Delay3/1
  Sqrt2/1 -> Switch/2, Switch1/2
  PF-Statik/1 -> Sum4/2
  P Filter Init/1(dP) -> Sum5/1
  [Ta] -> Divide3/1
  [phi0] -> Integrator (Angle)/3(d_phi0)
  Sum8/1 -> P Filter Init/2(dP0), Scope2/1, Sum5/2, Scope1/1
  sp_VSM/1 -> Bus Selector3/1, Bus Selector2/1
  Bus Selector3/1 -> Selector1/1  "<sp_PQ>"
  Integrator (Inertia)/1(omega [pu]) -> Sum3/2, omega0/1
  [Enable] -> Integrator (Inertia)/Enable
  Forward Damping/1 -> Sum1/2
  Saturation1/1 -> Mux/1, [E]
  omega0/1 -> [omega], Integrator (Angle)/2(omega)
  [Enable] -> Integrator (Angle)/1(Reset)
  [E0] -> Saturation/1
  Unit Delay2/1 -> Sum2/1
  [Tu] -> Q(U)-PI-Regler/1(Tau)
  [phi] -> Bus Creator3/4  "phi"
  Bus Selector13/6 -> [TPinit]  "<TPinit>"
  [E] -> Bus Creator3/5  "E"
  [ku] -> QU-Statik/2
  Sum2/1 -> Q(U)-PI-Regler/2(E)
  Data Type Conversion/1 -> [Enable]
  Unit Delay1/1 -> Subsystem/1(first_run)
  Constant2/1 -> Unit Delay1/1
  u_inv_dq/1 -> Subsystem/2(u_dq)
  [Enable] -> Detect Increase/1
  Param/1 -> Bus Selector13/1
  Bus Selector13/1 -> [Ta]  "<Ta>"
  Bus Selector13/2 -> [kpf]  "<kpf>"
  Bus Selector13/3 -> [kdf]  "<kdf>"
  Bus Selector13/4 -> [ku]  "<ku>"
  Bus Selector13/5 -> [Tu]  "<Tu>"
  [Enable] -> Logical Operator1/1
  Logical Operator1/1 -> P Filter Init/Enable
  Compare To Zero1/1 -> Logical Operator1/2
  [TPinit] -> Compare To Zero1/1, P Filter Init/1(Tau)
  Sum5/1 -> [d_P], Sum4/1
  Detect Increase/1 -> Subsystem/Enable
  Subsystem/2(u_ang) -> [phi0]
  Constant/1 -> Mux/2
  Mux/1 -> sp_u_inv_dq/1
  [pll_om] -> Integrator (Inertia)/2(omega0 [pu])
  Divide3/1 -> Integrator (Inertia)/1(dPTa)
  Bus Selector11/1 -> Selector3/1  "<vdq>"
  PQ_meas/1 -> Selector2/1
  [sp_VSM] -> Bus Creator3/6, Scope/1  "sp_VSM"
  omega3/1 -> Bus Creator3/3  "mdelta_f"
  omega2/1 -> Bus Creator3/2  "f"
  [d_omega] -> omega3/1
  omega1/1 -> [d_omega], Forward Damping/2
  [omega] -> omega2/1
  Bus Creator3/1 -> VSMdiag/1
  PLL/1 -> Bus Selector11/1
  Bus Selector2/1 -> 1/f1/1, Bus Creator/1  "<sp_f>"
  Sum3/1 -> omega1/1, PF-Statik/2
  Sum4/1 -> Divide3/2
  Sum1/1 -> phi_rad/1, [phi]  "Phi [rad]"
  [Enable] -> Bus Creator3/7  "VSM_enable"
  Selector3/1 -> Subsystem/3(u_dq_pll)
  Integrator (Angle)/1(phi) -> Sum1/1, Scope3/1
  Bus Selector11/3 -> 1/f3/1  "<f>"
  1/f3/1 -> [pll_om]
  [kdf] -> Forward Damping/1
  [kpf] -> PF-Statik/1
  "PQ_meas "/1 -> Selector5/1
  Bus Selector1/2 -> Selector6/1  "<sp_PQ>"
  "sp_VSM "/1 -> Bus Selector1/1
  Sum6/1 -> [d_Q], QU-Statik/1
  Selector2/1 -> Sum8/1, Enabled Subsystem1/1(P)
  Mux1/1 -> Bus Creator3/1  "delta_PQ"
  [d_P] -> Mux1/1
  [d_Q] -> Mux1/2
  1/f1/1 -> Sum3/1
  Selector6/1 -> Sum6/1, Mux2/2
  Selector5/1 -> Sum6/2
  Bus Selector11/2 -> Subsystem/4(phi_pll)  "<phi>"
  [Enable] -> Q(U)-PI-Regler/Enable

== system AC_base_1_VSM_2_22a/Variant Subsystem1/VSM/VSM1/VSM/CONTROL/Virtual Circuit mit R und L/Current Predictor ==
  u : Inport
  Delay : Delay  DelayLength=1  InitialCondition=0
  Sum : Sum  Inputs=|-+
  Sum1 : Sum  Inputs=|++
  y : Outport
  wires:
  Sum1/1 -> y/1
  Sum/1 -> Sum1/1
  Delay/1 -> Sum/1
  u/1 -> Delay/1, Sum1/2, Sum/2

== system AC_base_1_VSM_2_22a/Variant Subsystem1/VSM/VSM1/VSM/CONTROL/Virtual Circuit mit R und L/PT1 ==
  U : Inport  SampleTime=Ts
  tau : Inport  Port=2  SampleTime=Ts
  Reset : Inport  Port=3  SampleTime=Ts
  Phi : Inport  Port=4
  Delay : Delay  DelayLength=1  InitialConditionSource=Input port  ExternalReset=Rising
      settings: InputPortMap=u0,r5,p4
  Divide : Product  Inputs=*/
  Gain : Gain  Gain=Ts
  Gain1 : Gain  Gain=K
  Saturation : Saturate  UpperLimit=inf  LowerLimit=Ts
  Sum : Sum  Inputs=|++
  Sum2 : Sum  Inputs=|+-
  Unit Delay2 : UnitDelay  InitialCondition=[0 0 0]  SampleTime=ControlSampleTime  HasFrameUpgradeWarning=on
  dq0->ab0 phi : FriedrichLibrary/Transformations/dq0->ab0 phi  SystemSampleTime=-1  VariantActivationTime=update diagram  Latency=0  AutoFrameSizeCalculation=off
  Y : Outport
  wires:
  dq0->ab0 phi/1 -> Delay/3
  Gain1/1 -> Y/1
  Sum2/1 -> Gain/1
  U/1 -> Sum2/1
  Gain/1 -> Divide/1
  Delay/1 -> Sum/2, Sum2/2
  tau/1 -> Saturation/1
  Divide/1 -> Sum/1
  Saturation/1 -> Divide/2
  Reset/1 -> Delay/2
  Sum/1 -> Delay/1, Unit Delay2/1, Gain1/1
  Unit Delay2/1 -> dq0->ab0 phi/1
  Phi/1 -> dq0->ab0 phi/2

== system AC_base_1_VSM_2_22a/Variant Subsystem1/VSM/VSM1/VSM/CONTROL/Virtual Circuit mit R und L/PT2 ==
  U : Inport  SampleTime=Ts
  tau : Inport  Port=2  SampleTime=Ts
  Reset : Inport  Port=3  SampleTime=Ts
  Phi : Inport  Port=4
  Delay : Delay  DelayLength=1  InitialConditionSource=Input port  ExternalReset=Rising
      settings: InputPortMap=u0,r5,p4
  Divide : Product  Inputs=*/
  Gain : Gain  Gain=Ts
  Gain1 : Gain  Gain=K
  Saturation : Saturate  UpperLimit=inf  LowerLimit=Ts
  Sum : Sum  Inputs=|++
  Sum2 : Sum  Inputs=|+-
  Unit Delay2 : UnitDelay  InitialCondition=[0 0 0]  SampleTime=ControlSampleTime  HasFrameUpgradeWarning=on
  dq0->ab0 phi1 : FriedrichLibrary/Transformations/dq0->ab0 phi  SystemSampleTime=-1  VariantActivationTime=update diagram  Latency=0  AutoFrameSizeCalculation=off
  Y : Outport
  wires:
  Phi/1 -> dq0->ab0 phi1/2
  Unit Delay2/1 -> dq0->ab0 phi1/1
  Sum/1 -> Gain1/1, Unit Delay2/1, Delay/1
  Reset/1 -> Delay/2
  Saturation/1 -> Divide/2
  Divide/1 -> Sum/1
  tau/1 -> Saturation/1
  Delay/1 -> Sum2/2, Sum/2
  Gain/1 -> Divide/1
  U/1 -> Sum2/1
  Sum2/1 -> Gain/1
  Gain1/1 -> Y/1
  dq0->ab0 phi1/1 -> Delay/3

== system AC_base_1_VSM_2_22a/Variant Subsystem1/VSM/VSM1/VSM/CONTROL/Virtual Circuit1/Current Predictor ==
  u : Inport
  Delay : Delay  DelayLength=1  InitialCondition=0
  Sum : Sum  Inputs=|-+
  Sum1 : Sum  Inputs=|++
  y : Outport
  wires:
  Sum1/1 -> y/1
  Sum/1 -> Sum1/1
  Delay/1 -> Sum/1
  u/1 -> Delay/1, Sum1/2, Sum/2

== system AC_base_1_VSM_2_22a/Variant Subsystem1/VSM/VSM1/VSM/CONTROL/Virtual Circuit1/PT1 ==
  U : Inport  SampleTime=Ts
  tau : Inport  Port=2  SampleTime=Ts
  Reset : Inport  Port=3  SampleTime=Ts
  Delay : Delay  DelayLength=1
  Divide : Product  Inputs=*/
  Gain : Gain  Gain=Ts
  Gain1 : Gain  Gain=K
  Saturation : Saturate  UpperLimit=inf  LowerLimit=Ts
  Sum : Sum  Inputs=|++
  Sum2 : Sum  Inputs=|+-
  Switch : Switch  Criteria=u2 > Threshold  SaturateOnIntegerOverflow=off  InputSameDT=off
  Y : Outport
  wires:
  Sum/1 -> Switch/3
  Switch/1 -> Delay/1, Gain1/1
  Gain1/1 -> Y/1
  Sum2/1 -> Gain/1
  U/1 -> Sum2/1, Switch/1
  Gain/1 -> Divide/1
  Delay/1 -> Sum/2, Sum2/2
  tau/1 -> Saturation/1
  Divide/1 -> Sum/1
  Saturation/1 -> Divide/2
  Reset/1 -> Switch/2

== system AC_base_1_VSM_2_22a/Variant Subsystem1/VSM/VSM1/VSM/CONTROL/Virtual Circuit1/PT2 ==
  U : Inport  SampleTime=Ts
  tau : Inport  Port=2  SampleTime=Ts
  Reset : Inport  Port=3  SampleTime=Ts
  Phi : Inport  Port=4
  Delay : Delay  DelayLength=1  InitialConditionSource=Input port  ExternalReset=Rising
      settings: InputPortMap=u0,r5,p4
  Divide : Product  Inputs=*/
  Gain : Gain  Gain=Ts
  Gain1 : Gain  Gain=K
  Saturation : Saturate  UpperLimit=inf  LowerLimit=Ts
  Sum : Sum  Inputs=|++
  Sum2 : Sum  Inputs=|+-
  Unit Delay2 : UnitDelay  InitialCondition=[0 0 0]  SampleTime=ControlSampleTime  HasFrameUpgradeWarning=on
  dq0->ab0 phi1 : FriedrichLibrary/Transformations/dq0->ab0 phi  SystemSampleTime=-1  VariantActivationTime=update diagram  Latency=0  AutoFrameSizeCalculation=off
  Y : Outport
  wires:
  Phi/1 -> dq0->ab0 phi1/2
  Unit Delay2/1 -> dq0->ab0 phi1/1
  Sum/1 -> Gain1/1, Unit Delay2/1, Delay/1
  Reset/1 -> Delay/2
  Saturation/1 -> Divide/2
  Divide/1 -> Sum/1
  tau/1 -> Saturation/1
  Delay/1 -> Sum2/2, Sum/2
  Gain/1 -> Divide/1
  U/1 -> Sum2/1
  Sum2/1 -> Gain/1
  Gain1/1 -> Y/1
  dq0->ab0 phi1/1 -> Delay/3

== system AC_base_1_VSM_2_22a/Variant Subsystem1/VSM/VSM1/VSM/CONTROL/i_dq_ctrl/PI ==
  di : Inport
  u0 : Inport  Port=2
  Enable : EnablePort  StatesWhenEnabling=reset
  Gain4 : Gain  Gain=Ki
  Gain5 : Gain  Gain=Kp
  Integrator (inertia) : DiscreteIntegrator  gainval=1  InitialConditionSource=external  InitialCondition=1  SampleTime=ControlSampleTime  ICPrevOutput=DiscIntNeverNeededParam  ICPrevScaledInput=DiscIntNeverNeededParam
  Product : Product
  Product1 : Product
  Step : Step  Time=8  Before=1  SampleTime=0
  Step1 : Step  Time=8.05+10  Before=1  After=0.1  SampleTime=0
  Sum2 : Sum  Inputs=++|
  u : Outport  VectorParamsAs1DForOutWhenUnconnected=off
  wires:
  Step1/1 -> Product1/1
  Step/1 -> Product/1
  Product/1 -> Sum2/1
  Product1/1 -> Integrator (inertia)/1
  Gain4/1 -> Product1/2
  Gain5/1 -> Product/2
  Integrator (inertia)/1 -> Sum2/2
  di/1 -> Gain5/1, Gain4/1
  Sum2/1 -> u/1
  u0/1 -> Integrator (inertia)/2

== system AC_base_1_VSM_2_22a/Variant Subsystem1/VSM/VSM1/VSM/MANAGEMENT/Subsystem1/Enabled Subsystem ==
  i_abs : Inport
  i_pq : Inport  Port=2
  Enable : EnablePort
  i abs_pre : Outport
  i_pq_pre : Outport  Port=2
  wires:
  i_pq/1 -> i_pq_pre/1
  i_abs/1 -> i abs_pre/1

== system AC_base_1_VSM_2_22a/Variant Subsystem1/VSM/VSM1/VSM/MANAGEMENT/Subsystem1/Subsystem ==
  note: zweiter Faktor bei clearing für richtiges Q
      |
      | bei Eintritt mit Halten aber fester Grenze
      |
      | bis jetzt über Zeit abgeschaltet bei clearing ohne Halten
  note: für mean muss simscape installiert sein
  i_inv : Inport
  PQ_out : Inport  Port=2
  iabs : Inport  Port=3
  U_cap : Inport  Port=4
  PQ_pre : Inport  Port=5
  i abs_pre : Inport  Port=6
  angle_i : Inport  Port=7
  Enable : EnablePort
  Abs : Abs  SaturateOnIntegerOverflow=off
  Add : Sum  Inputs=+-
  Clock : Clock
  Complex to Magnitude-Angle : ComplexToMagnitudeAngle
  Demux1 : Demux  Outputs=2
  Discrete Derivative2 : simulink/Discrete/Discrete Derivative  gainval=1.0  ICPrevScaledInput=0.0  OutMin=[]  OutMax=[]  OutDataType=fixdt(1, 16)  OutScaling=2^-10  DoSatur=off
  Discrete-Time Integrator : DiscreteIntegrator  SampleTime=-1  ICPrevOutput=DiscIntNeverNeededParam  ICPrevScaledInput=DiscIntNeverNeededParam
  Divide2 : Product  Inputs=*/
  Gain : Gain  Gain=1000  SaturateOnIntegerOverflow=on  OutDataTypeStr=Inherit: Same as input  ParamDataTypeStr=Inherit: Same as input
  K1 : Constant  Value=1./1000  SampleTime=Ts
  MATLAB Function1 : MATLAB Function  TreatAsAtomicUnit=on  SystemSampleTime=ControlSampleTime
  MATLAB Function2 : MATLAB Function  Commented=on  TreatAsAtomicUnit=on  SystemSampleTime=ControlSampleTime
  Memory : Memory
  Real-Imag to Complex : RealImagToComplex
  Relational Operator : RelationalOperator  OutDataTypeStr=boolean  ZeroCross=off  SampleTime=Ts  InputSameDT=off
  Scope1 : Scope  NumInputPorts=2
  Scope2 : Scope  NumInputPorts=2
  Selector3 : Selector  InputPortWidth=2  IndexOptions=Index vector (dialog)  Indices=2  OutputSizes=1
  Signal Specification9 : SignalSpecification  Dimensions=[1 2]
  Sum : Sum  Inputs=+-  InputSameDT=on  SaturateOnIntegerOverflow=on  OutDataTypeStr=Inherit: Same as first input
  Switch : Switch  Threshold=0.5  SaturateOnIntegerOverflow=off
  Transport Delay : TransportDelay  DelayTime=0.002
  Transport Delay1 : TransportDelay  DelayTime=1./1000  BufferSize=2048*4  PadeOrder=2
  i_sp : Outport
  CC : Outport  Port=2
  set : Outport  Port=3
  wires:
  Switch/1 -> Memory/1, Scope2/2, MATLAB Function1/4(der)
  Abs/1 -> Discrete-Time Integrator/1
  Transport Delay1/1 -> Sum/2
  K1/1 -> Relational Operator/2
  Clock/1 -> Relational Operator/1
  Gain/1 -> Switch/1
  Sum/1 -> Gain/1
  Discrete-Time Integrator/1 -> Transport Delay1/1, Sum/1
  Memory/1 -> Switch/3
  Relational Operator/1 -> Switch/2
  Signal Specification9/1 -> i_sp/1
  angle_i/1 -> MATLAB Function1/10(angle_i)
  Real-Imag to Complex/1 -> Complex to Magnitude-Angle/1
  Demux1/2 -> Real-Imag to Complex/2
  Complex to Magnitude-Angle/2 -> MATLAB Function1/9(angle_pre)
  PQ_pre/1 -> Demux1/1, MATLAB Function1/6(i_pq_pre)
  Demux1/1 -> Real-Imag to Complex/1
  Selector3/1 -> Discrete Derivative2/1
  Divide2/1 -> Scope2/1, Selector3/1
  MATLAB Function1/3(set1) -> Scope1/1, set/1
  Discrete Derivative2/1 -> Abs/1
  i_inv/1 -> MATLAB Function1/1(i_inv)
  Add/1 -> MATLAB Function1/8(u_diff)
  Transport Delay/1 -> Add/2
  i abs_pre/1 -> MATLAB Function1/7(i_abs_pre)
  MATLAB Function1/2(CC) -> CC/1
  MATLAB Function1/1(i_sp) -> Signal Specification9/1
  U_cap/1 -> Transport Delay/1, Add/1, Divide2/2, MATLAB Function1/5(U_cap)
  iabs/1 -> MATLAB Function1/3(i_abs)
  PQ_out/1 -> Divide2/1, MATLAB Function1/2(PQ_out)

== system AC_base_1_VSM_2_22a/Variant Subsystem1/VSM/VSM1/VSM/MANAGEMENT/sp_VSM/E(PQ) ==
  E : Inport
  cmd : Inport  Port=2
  sp_PQ : Inport  Port=3
  Abs : Abs  SaturateOnIntegerOverflow=off
  Add : Sum
  Add1 : Sum  Inputs=--
  Add2 : Sum  Inputs=+++
  Bus Selector : BusSelector  OutputSignals=Param.VC.R1,Param.VC.R1t,Param.VC.L1,Param.VC.L1t,Param.VSM.ku
  Bus Selector1 : BusSelector  OutputSignals=Param.VSM.sp_E_comp
  Constant : Constant
  Demux : Demux  Outputs=2
  Display{,1..4} (5 alike) : Display
  Divide : Product  Inputs=/*
  Product : Product
  Product1 : Product
  Real-Imag to Complex : RealImagToComplex
  Real-Imag to Complex1 : RealImagToComplex
  Switch : Switch  Criteria=u2 ~= 0  SaturateOnIntegerOverflow=off  InputSameDT=off
  "cmd " : InportShadow  Port=2
  sp_E : Outport  VectorParamsAs1DForOutWhenUnconnected=off
  wires:
  Constant/1 -> Add2/1, Divide/1
  Product1/1 -> Add2/3
  Bus Selector/5 -> Product1/2  "<ku>"
  Bus Selector1/1 -> Switch/2  "<sp_E_comp>"
  "cmd "/1 -> Bus Selector1/1
  Switch/1 -> sp_E/1
  cmd/1 -> Bus Selector/1
  Bus Selector/1 -> Add/1  "<R1>"
  Bus Selector/2 -> Add/2  "<R1t>"
  Bus Selector/3 -> Add1/1  "<L1>"
  Bus Selector/4 -> Add1/2  "<L1t>"
  Add/1 -> Real-Imag to Complex/1
  Add1/1 -> Real-Imag to Complex/2
  E/1 -> Switch/3
  sp_PQ/1 -> Demux/1
  Demux/1 -> Real-Imag to Complex1/1
  Demux/2 -> Real-Imag to Complex1/2, Product1/1
  Real-Imag to Complex1/1 -> Divide/2
  Divide/1 -> Product/1, Display/1  "current"
  Real-Imag to Complex/1 -> Product/2, Display1/1  "impedance"
  Product/1 -> Add2/2, Display2/1  "voltage"
  Abs/1 -> Switch/1, Display4/1
  Add2/1 -> Abs/1, Display3/1
